simulink model "ClosedLoopMotor"  (Simulink 8.6)
settings: Solver=ode4  StartTime=0.0  StopTime=0.5  FixedStep=1e-5  MaxStep=1e-3  RelTol=1e-3
values from neighbouring files (symbols this model uses):
  Dm = 90.9 * 10^-9    (= 9.09e-08)    [MotorConstants1624.m]    (also in MotorConstants1841.m)
  Jm = 0.68* (1/1000) * (1/100)^2    (= 6.8e-08)    [MotorConstants1624.m]    (also in MotorConstants1841.m = 8.5e-08)
  Kb = 0.555 * (1/1000)*1/(2*pi/60)    (= 0.00529985960496)    [MotorConstants1624.m]    (also in MotorConstants1841.m)
  Kemf = 9.55*(1/1000)    (= 0.00955)    [MotorConstants1841.m]
  Kn = 1800 *2*pi/60    (= 188.495559215)    [MotorConstants1624.m]    (also in MotorConstants1841.m)
  Kt = 5.30 * (1/1000)    (= 0.0053)    [MotorConstants1624.m]    (also in MotorConstants1841.m)
  Ktach = 1/(Kemf*Kn)    (= 0.555514635574)    [MotorConstants1841.m]
  La = 200* 10^-6    (= 0.0002)    [MotorConstants1624.m]    (also in MotorConstants1841.m)
  Ra = 9.1    [MotorConstants1624.m]    (also in MotorConstants1841.m)
libraries: dspsigops x1, simulink x1
settings Model: Creator=mrg  LastModifiedBy=Ngonie
settings DataIOCC: LimitDataPoints=off
settings DebuggingCC: FcnCallInpInsideContextMsg=UseLocalSettings
settings SFSimCC: SimParseCustomCode=off
settings GRTTargetCC: GeneratePreprocessorConditionals=Use local settings

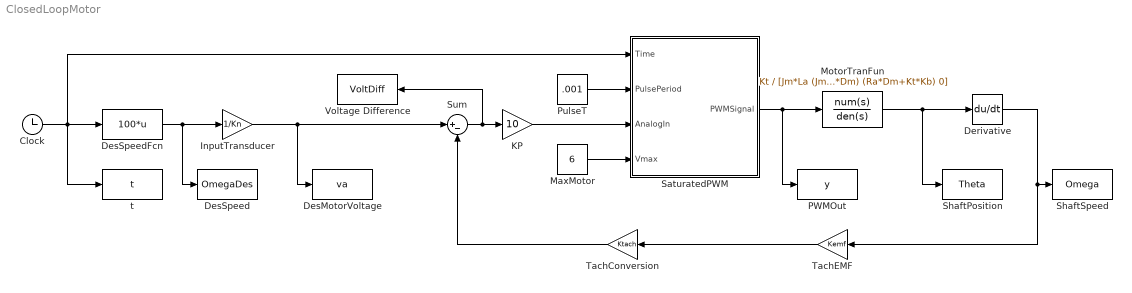
== system ClosedLoopMotor ==
  Clock : Clock
  Derivative : Derivative
  DesMotorVoltage : ToWorkspace  VariableName=va  SampleTime=-1
  DesSpeed : ToWorkspace  VariableName=OmegaDes  SampleTime=-1
  DesSpeedFcn : Fcn  Expr=100*u
  InputTransducer : Gain  Gain=1/Kn
  KP : Gain  Gain=10
  MaxMotor : Constant  Value=6
  MotorTranFun : TransferFcn  Numerator=Kt  Denominator=[Jm*La (Jm*Ra + La*Dm) (Ra*Dm+Kt*Kb) 0]
  PWMOut : ToWorkspace  VariableName=y  SampleTime=-1
  PulseT : Constant  Value=.001
  SaturatedPWM : Subsystem
  ShaftPosition : ToWorkspace  VariableName=Theta  SampleTime=-1
  ShaftSpeed : ToWorkspace  VariableName=Omega  SampleTime=-1
  Sum : Sum  Inputs=|+-
  TachConversion : Gain  Gain=Ktach
  TachEMF : Gain  Gain=Kemf
  Voltage Difference : ToWorkspace  VariableName=VoltDiff  SampleTime=-1
  t : ToWorkspace  VariableName=t  SampleTime=-1
  wires:
  Clock/1 -> DesSpeedFcn/1, t/1, SaturatedPWM/1(Time)
  DesSpeedFcn/1 -> InputTransducer/1, DesSpeed/1
  InputTransducer/1 -> DesMotorVoltage/1, Sum/1
  TachEMF/1 -> TachConversion/1
  TachConversion/1 -> Sum/2
  Derivative/1 -> ShaftSpeed/1, TachEMF/1
  MotorTranFun/1 -> Derivative/1, ShaftPosition/1
  SaturatedPWM/1(PWMSignal) -> PWMOut/1, MotorTranFun/1
  Sum/1 -> KP/1, Voltage Difference/1
  PulseT/1 -> SaturatedPWM/2(PulsePeriod)
  KP/1 -> SaturatedPWM/3(AnalogIn)
  MaxMotor/1 -> SaturatedPWM/4(Vmax)

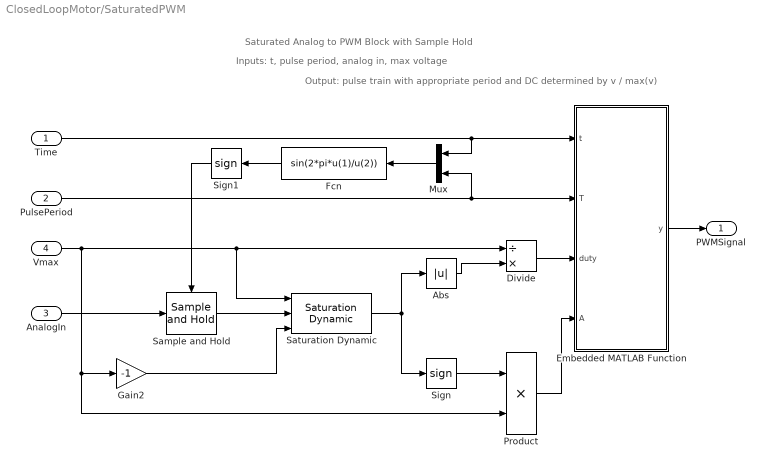
== system ClosedLoopMotor/SaturatedPWM ==
  note: Saturated Analog to PWM Block with Sample Hold
  note: Inputs: t, pulse period, analog in, max voltage
  note: Output: pulse train with appropriate period and DC determined by v / max(v)
  Time : Inport
  PulsePeriod : Inport  Port=2
  AnalogIn : Inport  Port=3
  Vmax : Inport  Port=4
  Abs : Abs
  Divide : Product  Inputs=/*
  Embedded MATLAB Function : MATLAB Function  TreatAsAtomicUnit=on
  Fcn : Fcn  Expr=sin(2*pi*u(1)/u(2))
  Gain2 : Gain  Gain=-1
  Mux : Mux  Inputs=2
  Product : Product  RndMeth=Zero
  Sample and Hold : dspsigops/Sample and Hold  trig=Rising edge  initCond=0  latchinput=off
  Saturation Dynamic : simulink/Discontinuities/Saturation Dynamic  OutMin=[]  OutMax=[]  OutDataTypeStr=Inherit: Same as second input  OutDataType=fixdt(1, 16)  OutScaling=2^-10  DoSatur=off
  Sign : Signum
  Sign1 : Signum
  PWMSignal : Outport
  wires:
  Time/1 -> Mux/1, Embedded MATLAB Function/1(t)
  PulsePeriod/1 -> Embedded MATLAB Function/2(T), Mux/2
  Embedded MATLAB Function/1(y) -> PWMSignal/1
  Gain2/1 -> Saturation Dynamic/3
  Vmax/1 -> Saturation Dynamic/1, Divide/1, Product/2, Gain2/1
  Saturation Dynamic/1 -> Sign/1, Abs/1
  Sign/1 -> Product/1
  Abs/1 -> Divide/2
  Divide/1 -> Embedded MATLAB Function/3(duty)
  Fcn/1 -> Sign1/1
  Mux/1 -> Fcn/1
  Product/1 -> Embedded MATLAB Function/4(A)
  Sign1/1 -> Sample and Hold/Trigger
  AnalogIn/1 -> Sample and Hold/1
  Sample and Hold/1 -> Saturation Dynamic/2

== matlab function SaturatedPWM/Embedded MATLAB Function ==
  data: t input double; y output double; T input double; duty input double; A input double
function y = fcn(t, T, duty, A)

y = A*(mod(t, T)<(duty*T));
